simulink model "busobject"  (Simulink 6.6)
settings: Solver=FixedStepDiscrete  StartTime=0.0  StopTime=10.0  FixedStep=1  RelTol=1e-3
PreLoadFcn:
  | busobjectspec
settings Model: Creator=hnine  LastModifiedBy=hnine
settings DataIOCC: SaveFormat=Structure

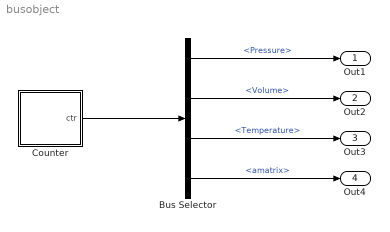
== system busobject ==
  Bus Selector : BusSelector  OutputSignals=environment.Pressure,environment.Volume,environment.Temperature,amatrix
  Counter : Stateflow chart
  Out1 : Outport
  Out2 : Outport  Port=2
  Out3 : Outport  Port=3
  Out4 : Outport  Port=4
  wires:
  Counter/1(ctr) -> Bus Selector/1
  Bus Selector/1 -> Out1/1  "<Pressure>"
  Bus Selector/2 -> Out2/1  "<Volume>"
  Bus Selector/3 -> Out3/1  "<Temperature>"
  Bus Selector/4 -> Out4/1  "<amatrix>"

== stateflow chart Counter ==
  state s1
  (default) -> s1 : / ctr.environment.Pressure = 1; ctr.environment.Temperature = 2; ctr.environment.Volume = 0; ctr.amatrix = 0;
  s1 -> s1 [order 1] : [ctr.environment.Volume < 4] /
      | ctr.environment.Volume = ctr.environment.Volume+1;
      | ctr.environment.Pressure = ctr.environment.Pressure+1;
      | ctr.environment.Temperature = ctr.environment.Temperature+1;
      | ctr.amatrix = 1;
  s1 -> s1 [order 2] : [ctr.environment.Volume >= 4] /
      | ctr.environment.Volume = 0;
      | ctr.environment.Pressure = 1;
      | ctr.environment.Temperature = 2;
      | ctr.amatrix = 2;
  data: ctr output boprimary =1
